simulink model "WaterTank_model"  (R2024b)
settings: Solver=FixedStepAuto  StartTime=0.0  StopTime=10.0  RelTol=1e-3
undefined symbols (not defined in the file): InitialHeight, InputFlowRate, MaxVoltage, MinVoltage, OutputFlowRate, TankArea
settings Model: Creator=felipe  LastModifiedBy=felipe
settings OptimizationCC: PassReuseOutputArgsAs=Individual arguments  OptimizeBlockOrder=speed  DifferentSizesBufferReuse=on  EfficientTunableParamExpr=on
settings DebuggingCC: ParameterTunabilityLossMsg=error
settings HardwareCC: TargetBitPerLong=64  TargetBitPerPointer=64  TargetBitPerSizeT=64  TargetBitPerPtrDiffT=64  TargetLongLongMode=on  TargetIntDivRoundTo=Zero  TargetEndianess=LittleEndian  TargetWordSize=64  TargetHWDeviceType=MATLAB Host  ProdEqTarget=off
settings SFSimCC: MATLABDynamicMemAlloc=off
settings RTWCC: Description=Embedded Coder (host-based shared library target)  SystemTargetFile=ert_shrlib.tlc  TemplateMakefile=ert_default_tmf  RTWVerbose=off
settings RTWCC: CustomSourceCode=|
  | #define CONCAT(str1, str2, str3) CONCAT_(str1, str2, str3)
  | #define CONCAT_(str1, str2, str3) str1 ## str2 ## str3
  | #define GET_MMI_FUNC    CONCAT(MODEL  , _GetCAPImmi ,  )
  | #define RT_MODEL_STRUCT CONCAT(RT_MODEL_ , MODEL  , _T )
  | 
  | void* GET_MMI_FUNC(void* voidPtrToRealTimeStructure)
  | {
  | rtwCAPI_ModelMappingInfo* mmiPtr = &(rtmGetDataMapInfo( ( RT_MODEL_STRUCT * )(voidPtrToRealTimeStructure) ).mmi);
  | return (void*) mmiPtr;
  | }
settings CodeAppCC: GenerateComments=off  IgnoreCustomStorageClasses=off  OperatorAnnotations=on  SimulinkDataObjDesc=on  SFDataObjDesc=on  SimulinkBlockComments=off
settings STFCustomTargetCC: TargetLangStandard=C99 (ISO)  MultiwordLength=256  ParMdlRefBuildCompliant=on  CompOptLevelCompliant=on  IncludeMdlTerminateFcn=off  CombineOutputUpdateFcns=on  CombineSignalStateStructs=on  SuppressErrorStatus=on  ERTCustomFileBanners=on  SupportAbsoluteTime=off  CodeInterfacePackaging=Reusable function  SupportComplex=off  SupportContinuousTime=off  SupportNonInlinedSFcns=off  RemoveResetFunc=on  MATLABClassNameForMDSCustomization=Simulink.SoftwareTarget.ERTCustomization  ModelStepFunctionPrototypeControlCompliant=on  GenerateAllocFcn=on  UseToolchainInfoCompliant=on  SystemTargetFile=ert_shrlib.tlc
settings ERTTargetCC: TargetLangStandard=C99 (ISO)  ConcurrentExecutionCompliant=off  IncludeMdlTerminateFcn=off  CombineSignalStateStructs=on  SuppressErrorStatus=on  SupportAbsoluteTime=off  CodeInterfacePackaging=Reusable function  SupportComplex=off  CPPClassGenCompliant=off  GenerateAllocFcn=on  InlinedParameterPlacement=Hierarchical  RootIOFormat=Part of model data structure  RTWCAPIParams=on  RTWCAPIRootIO=on  ERTCustomFileTemplate=example_file_process.tlc

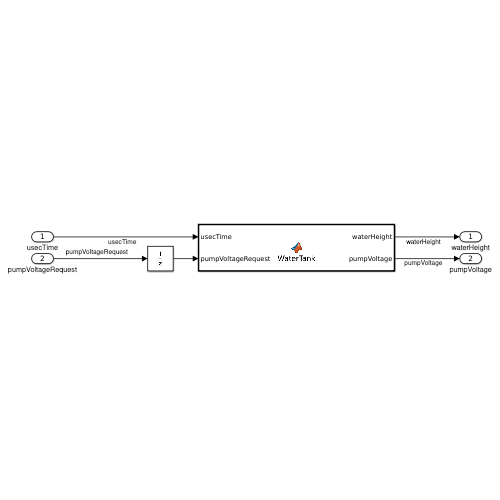
[thumbnail: Simulink's stored preview of the top-level diagram]
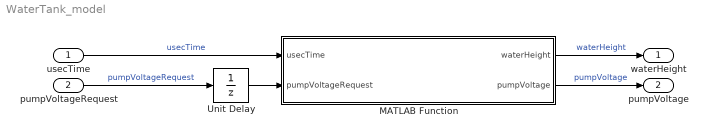
== system WaterTank_model ==
  usecTime : Inport
  pumpVoltageRequest : Inport  Port=2
  MATLAB Function : MATLAB Function  TreatAsAtomicUnit=on
  Unit Delay : UnitDelay  SampleTime=-1  HasFrameUpgradeWarning=on
  waterHeight : Outport
  pumpVoltage : Outport  Port=2
  wires:
  pumpVoltageRequest/1 -> Unit Delay/1  "pumpVoltageRequest"
  usecTime/1 -> MATLAB Function/1(usecTime)  "usecTime"
  MATLAB Function/1(waterHeight) -> waterHeight/1  "waterHeight"
  Unit Delay/1 -> MATLAB Function/2(pumpVoltageRequest)
  MATLAB Function/2(pumpVoltage) -> pumpVoltage/1  "pumpVoltage"

== matlab function WaterTank_model/MATLAB Function ==
  data: usecTime input; waterHeight output; pumpVoltageRequest input size=1; MaxVoltage parameter; pumpVoltage output; MinVoltage parameter; InitialHeight parameter; InputFlowRate parameter; OutputFlowRate parameter; TankArea parameter
function [waterHeight,pumpVoltage] = WaterTank(usecTime, pumpVoltageRequest, MaxVoltage, MinVoltage, InitialHeight, InputFlowRate, OutputFlowRate, TankArea)

% Persistent variables - these maintain their values after every call of
% the function
persistent lastHeight lastUsecTime
persistent aFlowRate bFlowRate tankArea
if isempty(lastHeight)
    % Initialization
    if MinVoltage < 0
        warning('WaterTank: MinVoltage is less than 0. Forcing it to 0.');
        MinVoltage = 0;
    end
    lastHeight = InitialHeight;
    lastUsecTime = 0.0;
    aFlowRate = OutputFlowRate; % m^{2.5}/s 
    bFlowRate = InputFlowRate; % 0.05 m³/s max
    tankArea = TankArea; % m² -> max height = 1.5 m
end

if pumpVoltageRequest < MinVoltage
    pumpVoltageRequest = MinVoltage;
elseif pumpVoltageRequest > MaxVoltage
    pumpVoltageRequest = MaxVoltage;
end

% Simple Euler method
waterHeight = ((pumpVoltageRequest * bFlowRate - (aFlowRate * sqrt(lastHeight)))/ tankArea) * (usecTime - lastUsecTime) * 1e-6 + lastHeight;

    if waterHeight < 0
        warning('WaterTank: Height is negative, setting to 0');
        waterHeight = 0;
    end

%  Update the last state
lastHeight = waterHeight;
lastUsecTime = usecTime;
pumpVoltage = pumpVoltageRequest;
end
